simulink model "SmallOffice_Atlanta_Occ_AL_testing"  (R2020a)
settings: Solver=FixedStepAuto  StartTime=186*86400  StopTime=191*86400  FixedStep=60  RelTol=1e-3
settings Model: Creator=zhelu  LastModifiedBy=yl3328

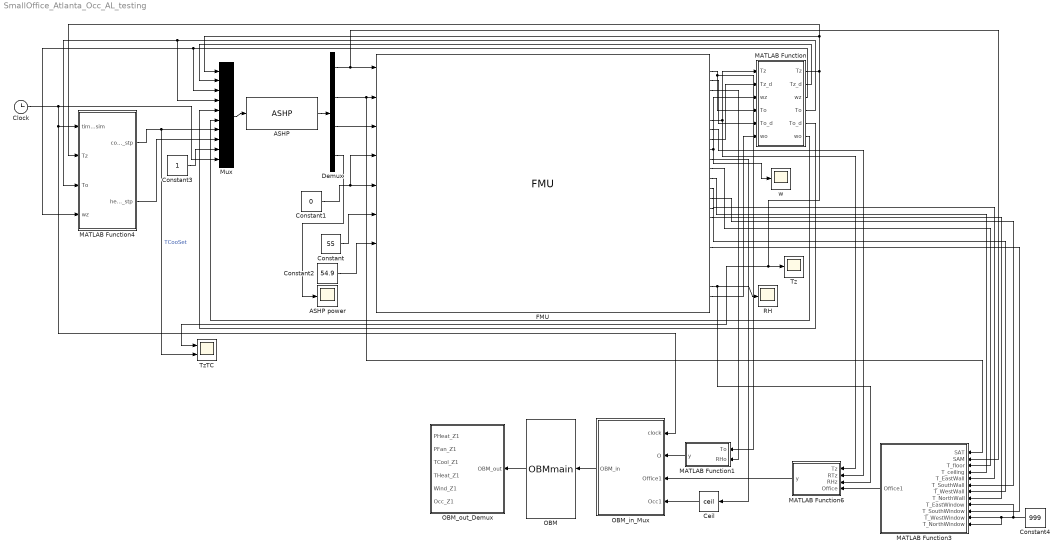
== system SmallOffice_Atlanta_Occ_AL_testing ==
  ASHP : M-S-Function  FunctionName=ASHP
  ASHP power : Scope
  Ceil : Rounding  Operator=ceil
  Clock : Clock
  Constant : Constant  Value=55
  Constant1 : Constant  Value=0
  Constant2 : Constant  Value=54.9
  Constant3 : Constant
  Constant4 : Constant  Value=999
  Demux : Demux
  FMU : FMU  FMUName=ASHRAE901_OfficeSmall_STD2004_Atlanta_5.fmu  FMUMode=CoSimulation
      mask Type: ASHRAE901_OfficeSmall_STD2004_Atlanta_5.idf [Co-Simulation, v2.0]
      mask Display:
      | disp('ASHRAE901_OfficeSmall_STD2004_Atlanta_5.idf');
      | port_label('output',1,'T_out');
      | port_label('output',2,'DewpointT_out');
      | port_label('output',3,'RH_out');
      | port_label('output',4,'Perimeter_ZN_1_SenLoads');
      | port_label('output',5,'Perimeter_ZN_1_LatLoads');
      | port_label('output',6,'Perimeter_ZN_1_Temp');
      | port_label('output',7,'Perimeter_ZN_1_RadTemp');
      | port_label('output',8,'Perimeter_ZN_1_DewpointT');
      | port_label('output',9,'Perimeter_ZN_1_HumdRat');
      | port_label('output',10,'Perimeter_ZN_1_Occ');
      | port_label('output',11,'Perimeter_ZN_1_FLOOR_T');
      | port_label('output',12,'Perimeter_ZN_1_CEILING_T');
      | port_label('output',13,'Perimeter_ZN_1_WALL_EAST_T');
      | port_label('output',14,'Perimeter_ZN_1_WALL_SOUTH_T');
      | port_label('output',15,'Perimeter_ZN_1_WALL_WEST_T');
      | port_label('output',16,'Perimeter_ZN_1_WALL_NORTH_T');
      | port_label('output',17,'Perimeter_ZN_1_WALL_SOUTH_WINDOW1_T');
      | port_label('output',18,'Perimeter_ZN_1_WALL_SOUTH_WINDOW2_T');
      | port_label('output',19,'Perimeter_ZN_1_WALL_SOUTH_WINDOW3_T');
      | port_label('output',20,'Perimeter_ZN_1_WALL_SOUTH_WINDOW4_T');
      | port_label('output',21,'Perimeter_ZN_1_WALL_SOUTH_WINDOW5_T');
      | port_label('output',22,'Perimeter_ZN_1_WALL_SOUTH_WINDOW6_T');
      | port_label('output',23,'Perimeter_ZN_1_RelaHumd');
      | port_label('output',24,'w_out');
      | port_label('input',1,'Perimeter_ZN_1 SupplyFlow');
      | port_label('input',2,'Perimeter_ZN_1 SupplyTemp');
      | port_label('input',3,'Perimeter_ZN_1 SupplyHumd');
      | port_label('input',4,'Perimeter_ZN_1_PHeat');
      | port_label('input',5,'Perimeter_ZN_1_PFan');
      | port_label('input',6,'Perimeter_ZN_1_TCool');
      | port_label('input',7,'Perimeter_ZN_1_THeat');
      | port_label('input',8,'OtherZN_TC');
      | port_label('input',9,'OtherZN_TH');
  MATLAB Function : MATLAB Function  TreatAsAtomicUnit=on
  MATLAB Function1 : MATLAB Function  TreatAsAtomicUnit=on
  MATLAB Function3 : MATLAB Function  TreatAsAtomicUnit=on
  MATLAB Function4 : MATLAB Function  TreatAsAtomicUnit=on
  MATLAB Function6 : MATLAB Function  TreatAsAtomicUnit=on
  Mux : Mux  Inputs=10
  OBM : M-S-Function  FunctionName=OBMmain
  OBM_in_Mux : MATLAB Function  TreatAsAtomicUnit=on
  OBM_out_Demux : MATLAB Function  TreatAsAtomicUnit=on
  RH : Scope
  Tz : Scope
  TzTC : Scope  NumInputPorts=2
  w : Scope
  wires:
  ASHP/1 -> Demux/1
  Constant2/1 -> FMU/7
  Constant/1 -> FMU/6
  Demux/1 -> MATLAB Function3/2(SAM), FMU/1
  Demux/2 -> MATLAB Function3/1(SAT), FMU/2
  Demux/3 -> FMU/3
  FMU/24 -> MATLAB Function/6("wo ")
  FMU/2 -> MATLAB Function/5("To_d ")
  FMU/1 -> MATLAB Function1/1(To), MATLAB Function/4("To ")
  FMU/8 -> MATLAB Function/2("Tz_d ")
  FMU/6 -> MATLAB Function6/1(Tz), MATLAB Function/1("Tz ")
  Constant1/1 -> FMU/4, FMU/5
  Constant3/1 -> Mux/9
  MATLAB Function4/2(heating_stp) -> Mux/8
  Mux/1 -> ASHP/1
  MATLAB Function/1(Tz) -> TzTC/1, Tz/1, MATLAB Function4/2(Tz), Mux/1
  MATLAB Function/2(Tz_d) -> Mux/2
  MATLAB Function/3(wz) -> MATLAB Function4/4(wz), Mux/3
  MATLAB Function/4(To) -> MATLAB Function4/3(To), Mux/4
  MATLAB Function/5(To_d) -> Mux/5
  MATLAB Function/6(wo) -> Mux/6
  Demux/4 -> ASHP power/1
  Clock/1 -> MATLAB Function4/1(time_sim), OBM_in_Mux/1(clock), Mux/10
  MATLAB Function4/1(cooling_stp) -> Mux/7, TzTC/2  "TCooSet"
  FMU/9 -> w/1, MATLAB Function/3("wz ")
  FMU/23 -> MATLAB Function6/3(RHz), RH/1
  OBM_in_Mux/1(OBM_in) -> OBM/1
  OBM/1 -> OBM_out_Demux/1(OBM_out)
  FMU/3 -> MATLAB Function1/2(RHo)
  MATLAB Function1/1(y) -> OBM_in_Mux/2(O)
  FMU/7 -> MATLAB Function6/2(RTz)
  MATLAB Function3/1(Office1) -> MATLAB Function6/4(Office)
  MATLAB Function6/1(y) -> OBM_in_Mux/3(Office1)
  FMU/10 -> Ceil/1
  Ceil/1 -> OBM_in_Mux/4(Occ1)
  FMU/11 -> MATLAB Function3/3(T_floor)
  FMU/12 -> MATLAB Function3/4(T_ceiling)
  FMU/13 -> MATLAB Function3/5(T_EastWall)
  FMU/14 -> MATLAB Function3/6(T_SouthWall)
  FMU/15 -> MATLAB Function3/7(T_WestWall)
  FMU/16 -> MATLAB Function3/8(T_NorthWall)
  Constant4/1 -> MATLAB Function3/9(T_EastWindow), MATLAB Function3/12(T_NorthWindow), MATLAB Function3/11(T_WestWindow)
  FMU/19 -> MATLAB Function3/10(T_SouthWindow)

== matlab function SmallOffice_Atlanta_Occ_AL_testing/MATLAB Function3 ==
  data: SAT input; SAM input; T_floor input; Office1 output; T_ceiling input; T_EastWall input; T_SouthWall input; T_WestWall input; T_NorthWall input; T_EastWindow input; T_SouthWindow input; T_WestWindow input; T_NorthWindow input
function Office1 = fcn(SAT,SAM,T_floor,T_ceiling,T_EastWall,T_SouthWall,T_WestWall,T_NorthWall,...
    T_EastWindow,T_SouthWindow,T_WestWindow,T_NorthWindow)
Office1=[SAT,SAM,T_floor,T_ceiling,T_EastWall,T_SouthWall,T_WestWall,T_NorthWall,...
    T_EastWindow,T_SouthWindow,T_WestWindow,T_NorthWindow];

== matlab function SmallOffice_Atlanta_Occ_AL_testing/MATLAB Function4 ==
  data: time_sim input; Tz input; To input; cooling_stp output; heating_stp output; wz input
function [cooling_stp,heating_stp]  = active_learning(time_sim,Tz,To,wz)
persistent cooling_stp_last
if isempty(cooling_stp_last)
    cooling_stp_last=0;
    cooling_stp_last=(78-32)/1.8;

end
cooling_stp = 0;

if mod(time_sim,86400)>5*3600 && mod(time_sim,86400)<20*3600
    if mod(time_sim,3600) == 0
        rng('shuffle');
        cooling_stp = 20+15*rand();
        cooling_stp_last=cooling_stp;
    else
        cooling_stp = cooling_stp_last;
    end
else
    cooling_stp=35;
end

heating_stp=cooling_stp-15;
end

== matlab function SmallOffice_Atlanta_Occ_AL_testing/MATLAB Function6 ==
  data: Tz input; y output; RTz input; RHz input; Office input
function y = fcn(Tz, RTz, RHz, Office)

y = [Tz, RTz, RHz, Office];

== matlab function SmallOffice_Atlanta_Occ_AL_testing/OBM_out_Demux ==
  data: OBM_out input; PHeat_Z1 output; PFan_Z1 output; TCool_Z1 output; THeat_Z1 output; Wind_Z1 output; Occ_Z1 output
function [PHeat_Z1,PFan_Z1,TCool_Z1,THeat_Z1,Wind_Z1,Occ_Z1] = fcn(OBM_out)

PHeat_Z1 = OBM_out(1);
PFan_Z1 = OBM_out(2);
TCool_Z1 = OBM_out(3);
THeat_Z1 = OBM_out(4);
Wind_Z1 = OBM_out(5);
Occ_Z1 = OBM_out(6);

== matlab function SmallOffice_Atlanta_Occ_AL_testing/OBM_in_Mux ==
  data: clock input; OBM_in output; O input; Office1 input; Occ1 input
function OBM_in = fcn(clock,O,Office1,Occ1)
% Assemble OBM inputs
OBM_in=[clock,O,Office1,Occ1]';

== matlab function SmallOffice_Atlanta_Occ_AL_testing/MATLAB Function ==
  data: Tz input; Tz output; Tz_d input; wz input; To input; To_d input; wo input; Tz_d output; wz output; To output; To_d output; wo output
function [Tz,Tz_d,wz,To,To_d,wo] = fcn(Tz,Tz_d,wz,To,To_d,wo)
Tz=Tz;
Tz_d=Tz_d;
wz=wz;
To=To;
To_d=To_d;
wo=wo;

== matlab function SmallOffice_Atlanta_Occ_AL_testing/MATLAB Function1 ==
  data: To input; y output; RHo input
function y = fcn(To,RHo)

y = [To RHo];
